simulink library "lib_square_root"  (R2023a)
settings: Solver=VariableStepAuto  StartTime=0.0  StopTime=10.0  RelTol=1e-3
undefined symbols (not defined in the file): lb_parLktInpData
libraries: lib_conversion x8, simulink x1
settings Model: Creator=cav2ofo  LastModifiedBy=lenovo
settings OptimizationCC: ReuseModelBlockBuffer=off

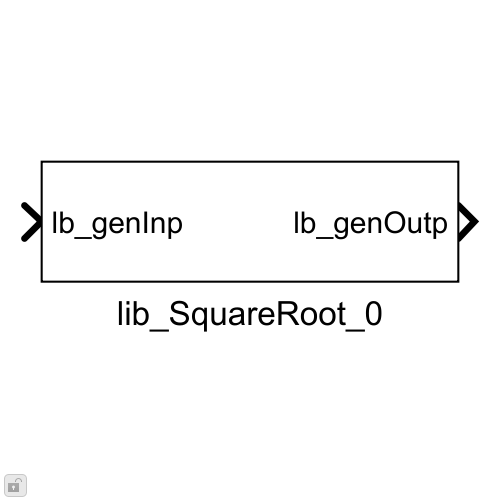
[thumbnail: Simulink's stored preview of the top-level diagram]
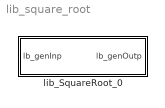
== system lib_square_root ==
  lib_SquareRoot_0 : Subsystem  mask{lb_parLktSize=128, lb_parInpDataType=uint16, lb_parOutpDataType=fixdt(0,16,2^-15,0)}
      mask prompts: lb_parLktSize "Look-up table size:"; lb_parInpDataType "Input data type:"; lb_parOutpDataType "Output data type:"
      mask init:
      | lb_parLktSizeNum = str2double(lb_parLktSize);
      | temp.lktInpData_vct = (0:1/(lb_parLktSizeNum-1):1);
      | lb_parLktOutpData = sqrt(temp.lktInpData_vct);
      | 
      | if ischar(lb_parInpDataType)
      |     lb_parSlopeSqrt = 1;
      |     if strcmp(lb_parInpDataType,'uint16')
      |         temp.inpDataTypeLen_scl = 16;
      |     else
      |         temp.inpDataTypeLen_scl = 32;
      |     end
      | else
      |     temp.inpDataTypeLen_scl = lb_parInpDataType.WordLength;
      |     lb_parSlopeSqrt = sqrt(lb_parInpDataType.Slope);
      | end
      | 
      | if temp.inpDataTypeLen_scl == 16
      |         lb_parNormFact = 2^16-1;        
      |         lb_parDataType1 = 'uint16';
      |         lb_parDataType2Len = 16;
      |         lb_parDataType2Prec = -7;      
      | else
      |         lb_parNormFact = 2^32-1;        
      |         lb_parDataType1 = 'uint32';
      |         lb_parDataType2Len = 32;
      |         lb_parDataType2Prec = -15;
      | end
      | lb_parNormFactSqrRoot = sqrt(lb_parNormFact);
      mask TypeOptions lb_parLktSize: 32 | 64 | 128 | 256 | 512 | 1024 | 2048 | 4096
      mask DialogControl DescGroupVar Prompt: VHIT control library
      mask DialogControl DescTextVar Prompt: Square root function
      mask DialogControl Container3 Prompt: Data type

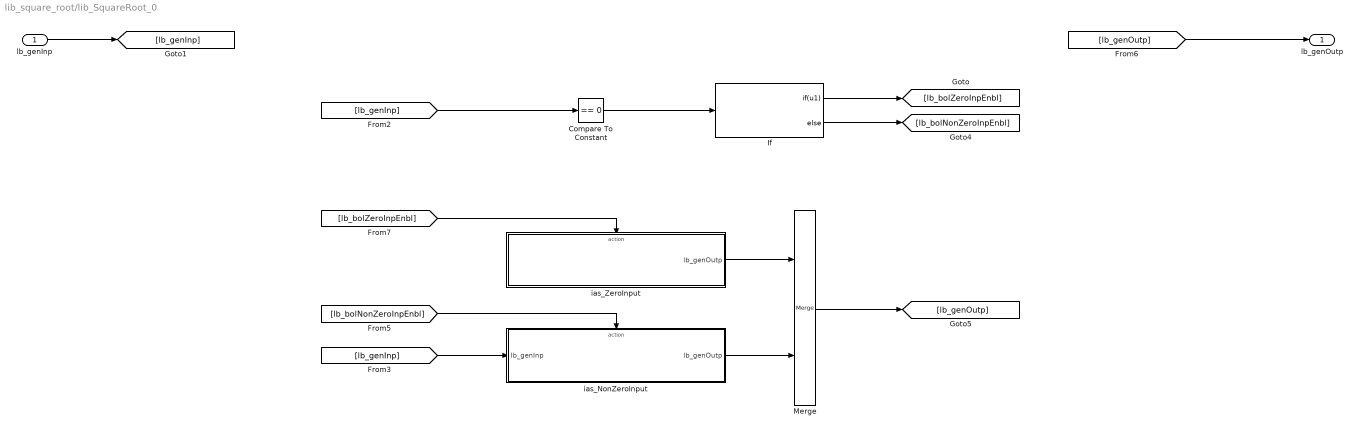
== system lib_square_root/lib_SquareRoot_0 ==
  lb_genInp : Inport
  Compare To Constant : simulink/Logic and Bit Operations/Compare To Constant  relop===  const=0  OutDataTypeStr=boolean
  If : If  IfExpression=u1
  Merge : Merge
  ias_NonZeroInput : Subsystem  TreatAsAtomicUnit=on
  ias_ZeroInput : Subsystem  TreatAsAtomicUnit=on
  lb_genOutp : Outport
  wires:
  Merge/1 -> [lb_genOutp]
  ias_NonZeroInput/1(lb_genOutp) -> Merge/2
  ias_ZeroInput/1(lb_genOutp) -> Merge/1
  [lb_bolNonZeroInpEnbl] -> ias_NonZeroInput/Action
  [lb_bolZeroInpEnbl] -> ias_ZeroInput/Action
  If/2 -> [lb_bolNonZeroInpEnbl]
  If/1 -> [lb_bolZeroInpEnbl]
  [lb_genInp] -> ias_NonZeroInput/1(lb_genInp)
  Compare To Constant/1 -> If/1
  [lb_genInp] -> Compare To Constant/1
  lb_genInp/1 -> [lb_genInp]
  [lb_genOutp] -> lb_genOutp/1

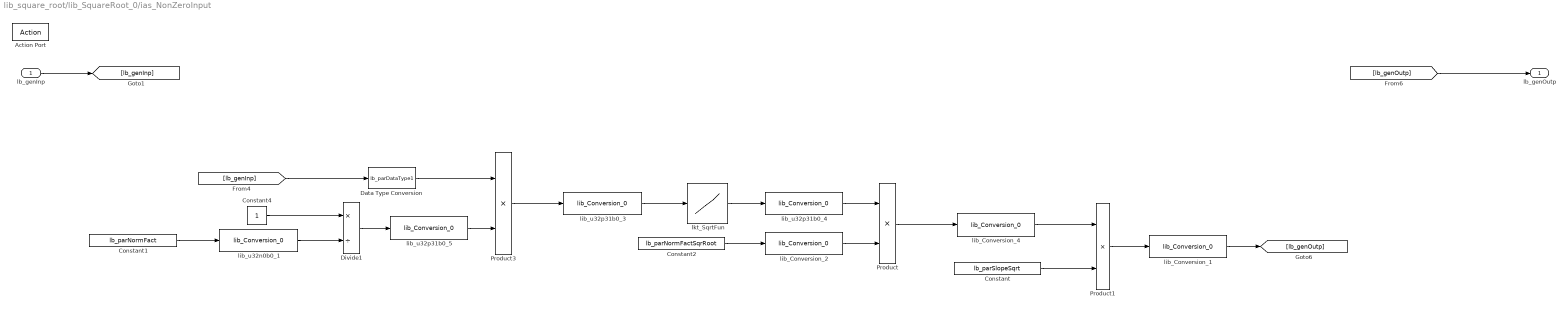
== system lib_square_root/lib_SquareRoot_0/ias_NonZeroInput ==
  lb_genInp : Inport
  Action Port : ActionPort
  Constant : Constant  Value=lb_parSlopeSqrt  OutDataTypeStr=fixdt(0,32,2^-31,0)
  Constant1 : Constant  Value=lb_parNormFact  OutDataTypeStr=Inherit: Inherit via back propagation
  Constant2 : Constant  Value=lb_parNormFactSqrRoot  OutDataTypeStr=Inherit: Inherit via back propagation
  Constant4 : Constant  OutDataTypeStr=uint32
  Data Type Conversion : DataTypeConversion  OutDataTypeStr=lb_parDataType1  ConvertRealWorld=Stored Integer (SI)  SaturateOnIntegerOverflow=off  RndMeth=Floor
  Divide1 : Product  Inputs=*/  OutDataTypeStr=fixdt(0,32,2^-31,0)
  Product : Product  OutDataTypeStr=Inherit: Inherit via back propagation  RndMeth=Simplest
  Product1 : Product  OutDataTypeStr=Inherit: Inherit via back propagation  RndMeth=Zero
  Product3 : Product  OutDataTypeStr=Inherit: Inherit via back propagation  RndMeth=Simplest
  lib_Conversion_1 : lib_conversion/lib_Conversion_0  lb_parDataType=lb_parOutpDataType  lb_parOutpMaxVal=[]  lb_parOutpMinVal=[]  lb_parSatFlag=off
  lib_Conversion_2 : lib_conversion/lib_Conversion_0  lb_parDataType=fixdt(0,lb_parDataType2Len,2^lb_parDataType2Prec,0)  lb_parOutpMaxVal=[]  lb_parOutpMinVal=[]  lb_parSatFlag=off
  lib_Conversion_4 : lib_conversion/lib_Conversion_0  lb_parDataType=fixdt(0,lb_parDataType2Len,2^lb_parDataType2Prec,0)  lb_parOutpMaxVal=[]  lb_parOutpMinVal=[]  lb_parSatFlag=off
  lib_u32n0b0_1 : lib_conversion/lib_Conversion_0  lb_parDataType=uint32  lb_parOutpMaxVal=[]  lb_parOutpMinVal=[]  lb_parSatFlag=off
  lib_u32p31b0_3 : lib_conversion/lib_Conversion_0  lb_parDataType=fixdt(0,32,2^-31,0)  lb_parOutpMaxVal=[]  lb_parOutpMinVal=[]  RndMeth=Simplest  lb_parSatFlag=off
  lib_u32p31b0_4 : lib_conversion/lib_Conversion_0  lb_parDataType=fixdt(0,32,2^-31,0)  lb_parOutpMaxVal=[]  lb_parOutpMinVal=[]  lb_parSatFlag=off
  lib_u32p31b0_5 : lib_conversion/lib_Conversion_0  lb_parDataType=fixdt(0,32,2^-31,0)  lb_parOutpMaxVal=[]  lb_parOutpMinVal=[]  RndMeth=Simplest  lb_parSatFlag=off
  lkt_SqrtFun : Lookup_n-D  NumberOfTableDimensions=1  BreakpointsSpecification=Even spacing  BreakpointsForDimension1=lb_parLktInpData  BreakpointsForDimension1FirstPoint=0  BreakpointsForDimension1Spacing=1/lb_parLktSizeNum  IndexSearchMethod=Evenly spaced points  BeginIndexSearchUsingPreviousIndexResult=on  Table=lb_parLktOutpData  ExtrapMethod=Clip  UseLastTableValue=on  InternalRulePriority=Speed  RndMeth=Simplest
  lb_genOutp : Outport
  wires:
  lib_u32p31b0_5/1 -> Product3/2
  Divide1/1 -> lib_u32p31b0_5/1
  lib_u32n0b0_1/1 -> Divide1/2
  Constant4/1 -> Divide1/1
  Product3/1 -> lib_u32p31b0_3/1
  [lb_genInp] -> Data Type Conversion/1
  Constant/1 -> Product1/2
  Product/1 -> lib_Conversion_4/1
  lib_Conversion_4/1 -> Product1/1
  Product1/1 -> lib_Conversion_1/1
  Constant2/1 -> lib_Conversion_2/1
  lkt_SqrtFun/1 -> lib_u32p31b0_4/1
  lib_Conversion_2/1 -> Product/2
  lib_u32p31b0_3/1 -> lkt_SqrtFun/1
  Data Type Conversion/1 -> Product3/1
  lib_Conversion_1/1 -> [lb_genOutp]
  Constant1/1 -> lib_u32n0b0_1/1
  lib_u32p31b0_4/1 -> Product/1
  lb_genInp/1 -> [lb_genInp]
  [lb_genOutp] -> lb_genOutp/1

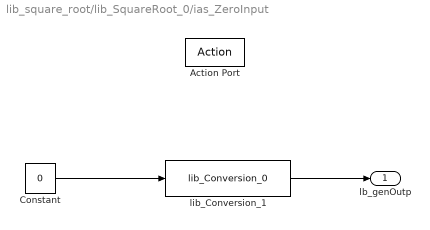
== system lib_square_root/lib_SquareRoot_0/ias_ZeroInput ==
  Action Port : ActionPort
  Constant : Constant  Value=0  OutDataTypeStr=Inherit: Inherit via back propagation
  lib_Conversion_1 : lib_conversion/lib_Conversion_0  lb_parDataType=lb_parOutpDataType  lb_parOutpMaxVal=[]  lb_parOutpMinVal=[]  lb_parSatFlag=off
  lb_genOutp : Outport
  wires:
  lib_Conversion_1/1 -> lb_genOutp/1
  Constant/1 -> lib_Conversion_1/1
